simulink model "StateSpace_from_ODE"  (R2022b)
settings: Solver=VariableStepAuto  StartTime=T_start  StopTime=T_stop  MaxStep=1e-1  RelTol=1e-3
undefined symbols (not defined in the file): alpha0, alpha1, beta0, gamma1, gamma2, u_cosA, u_cosO, u_expT, u_sinA, u_sinO, x1_0, x2_0
settings Model: Creator=fenu  LastModifiedBy=gianfrancofenu
settings DataIOCC: SaveFormat=Array  SaveState=on  SignalLogging=off  DSMLogging=off

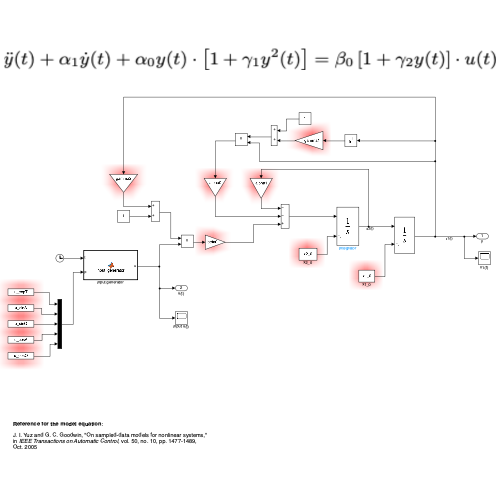
[thumbnail: Simulink's stored preview of the top-level diagram]
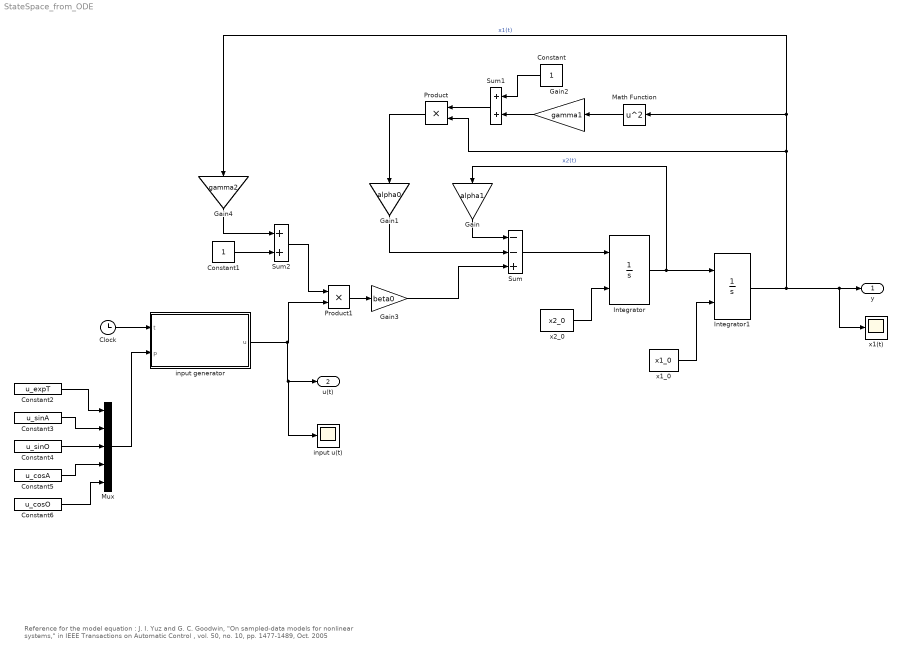
== system StateSpace_from_ODE ==
  note: Reference for the model equation :
      |
      | J. I. Yuz and G. C. Goodwin, "On sampled-data models for nonlinear systems," in IEEE Transactions on Automatic Control , vol. 50, no. 10, pp. 1477-1489, Oct. 2005
  Clock : Clock
  Constant : Constant  SampleTime=0
  Constant1 : Constant  SampleTime=0
  Constant2 : Constant  Value=u_expT  SampleTime=0
  Constant3 : Constant  Value=u_sinA  SampleTime=0
  Constant4 : Constant  Value=u_sinO  SampleTime=0
  Constant5 : Constant  Value=u_cosA  SampleTime=0
  Constant6 : Constant  Value=u_cosO  SampleTime=0
  Gain : Gain  Gain=alpha1
  Gain1 : Gain  Gain=alpha0
  Gain2 : Gain  Gain=gamma1
  Gain3 : Gain  Gain=beta0
  Gain4 : Gain  Gain=gamma2
  Integrator : Integrator  InitialConditionSource=external
  Integrator1 : Integrator  InitialConditionSource=external
  Math Function : Math  Operator=square
  Mux : Mux  Inputs=5
  Product : Product
  Product1 : Product
  Sum : Sum  Inputs=--+
  Sum1 : Sum
  Sum2 : Sum
  input generator : MATLAB Function  TreatAsAtomicUnit=on
  input u(t) : Scope
  x1(t) : Scope
  x1_0 : Constant  Value=x1_0  SampleTime=0
  x2_0 : Constant  Value=x2_0  SampleTime=0
  y : Outport
  u(t) : Outport  Port=2
  wires:
  Integrator/1 -> Integrator1/1, Gain/1  "x2(t)"
  x1_0/1 -> Integrator1/2
  x2_0/1 -> Integrator/2
  Integrator1/1 -> Product/2, Math Function/1, Gain4/1, x1(t)/1, y/1  "x1(t)"
  Sum/1 -> Integrator/1
  Gain/1 -> Sum/1
  Gain1/1 -> Sum/2
  Math Function/1 -> Gain2/1
  Gain2/1 -> Sum1/2
  Constant/1 -> Sum1/1
  Sum1/1 -> Product/1
  Product/1 -> Gain1/1
  Gain3/1 -> Sum/3
  Product1/1 -> Gain3/1
  Sum2/1 -> Product1/1
  Constant1/1 -> Sum2/2
  Gain4/1 -> Sum2/1
  Clock/1 -> input generator/1(t)
  input generator/1(u) -> input u(t)/1, u(t)/1, Product1/2
  Mux/1 -> input generator/2(p)
  Constant4/1 -> Mux/3
  Constant3/1 -> Mux/2
  Constant2/1 -> Mux/1
  Constant5/1 -> Mux/4
  Constant6/1 -> Mux/5

== matlab function StateSpace_from_ODE/input generator ==
  data: t input; u output; p input
function u = input_generator(t, p)
expT = p(1);
Asin = p(2);
OmSin = p(3);
Acos = p(4);
OmCos = p(5);
u = exp(-expT*t)*(Asin*sin(OmSin*t)-Acos*cos(OmCos*t));
